simulink model "Proyecto_Global_AyCD_Ultimo"  (R2017b)
settings: Solver=FixedStepAuto  StartTime=0.0  StopTime=inf  FixedStep=0.01  RelTol=1e-3  EnableMultiTasking=on
values from neighbouring files (symbols this model uses):
  AhMax = 1    [datosAyCD.m]
  AtMax = 1    [datosAyCD.m]
  Ba_b = zeros(1,60)    [PD_balanceo_CARGA_GainScheduling.m]
  Ba_h = Mh*n_h*Wpos_h    [PID_izaje_CARGA.m]
  Ba_t = Mt*n_t*Wpos_t    [PID_traslacion_CARRO.m]
  bContenedor = 2.5    [datosAyCD.m]
  bh = bhEq*rh^2/Rd^2    (= 28800)    [datosAyCD.m]
  bt = btEq*rt^2/Rw^2    (= 27000)    [datosAyCD.m]
  bw = 30000    [datosAyCD.m]
  cantidadCarrilesBarco = 9+1    (= 10)    [datosAyCD.m]
  g = 9.80665    [datosAyCD.m]
  hContenedor = 2.5    [datosAyCD.m]
  hLimInf = -17.5-2    (= -19.5)    [datosAyCD.m]
  hLimSup = 40+2    (= 42)    [datosAyCD.m]
  Kd = zeros(1,60)    [PD_balanceo_CARGA_AutoTunning.m]
  Kp = zeros(1,60)    [PD_balanceo_CARGA_AutoTunning.m]
  Ksa_b = zeros(1,60)    [PD_balanceo_CARGA_GainScheduling.m]
  Ksa_h = Mh*n_h*Wpos_h^2    [PID_izaje_CARGA.m]
  Ksa_t = Mt*n_t*Wpos_t^2    [PID_traslacion_CARRO.m]
  Ksia_h = Mh*Wpos_h^3    [PID_izaje_CARGA.m]
  Ksia_t = Mt*Wpos_t^3    [PID_traslacion_CARRO.m]
  Kw = 1800000    [datosAyCD.m]
  l1 = zeros(1,60)    [PD_balanceo_CARGA_AutoTunning.m]
  Mh = (Jd+Jmh*rh^2) / (Rd^2)    (= 48014.2222222)    [datosAyCD.m]
  mlMax = mlMin+48000    (= 65000)    [datosAyCD.m]
  mlVacio = 15000    [datosAyCD.m]
  Mt = mc + (Jw+Jmt*rt^2) / (Rw^2)    (= 59008)    [datosAyCD.m]
  nRand = [14 17 20 22 20 17 14 8 8 8]    [datosAyCD.m]
  Rd = 0.75    [datosAyCD.m]
  rh = 30    [datosAyCD.m]
  rt = 15    [datosAyCD.m]
  Rw = 0.5    [datosAyCD.m]
  Tf = zeros(1,60)    [PD_balanceo_CARGA_AutoTunning.m]
  tLimDer = 50+2    (= 52)    [datosAyCD.m]
  tLimIzq = -30-2    (= -32)    [datosAyCD.m]
  VhMaxC = 1.5    [datosAyCD.m]
  VhMaxV = 3    [datosAyCD.m]
  xCarrilBarco = zeros(1,cantidadCarrilesBarco)    [datosAyCD.m]
  xCarrilMuelle = [-30,-25,-20,-15,-10,-5]    [datosAyCD.m]
  yCarrilBarcoPar = zeros(1,cantidadCarrilesBarco)    [datosAyCD.m]
  ySB = 15    [datosAyCD.m]
  yt0 = 45    [datosAyCD.m]
undefined symbols (not defined in the file or in its folder): carrilObjetivoInput, carrilPartidaInput, lh
libraries: simulink x5
settings Model: Creator=Facundo  LastModifiedBy=Martin Da Corta
settings DataIOCC: LimitDataPoints=on
settings OptimizationCC: LifeSpan=inf
settings DebuggingCC: SFUnexpectedBacktrackingDiag=warning  SFNoUnconditionalDefaultTransitionDiag=warning  SFExecutionAtInitializationDiag=none
settings HardwareCC: ProdBitPerSizeT=32  ProdBitPerPtrDiffT=32  ProdWordSize=32  ProdHWDeviceType=Specified
settings ModelReferenceCC: PropagateSignalLabelsOutOfModel=off
settings RTWCC: TargetLang=C++
settings CodeAppCC: StateflowObjectComments=on
settings GRTTargetCC: TargetLangStandard=C89/C90 (ANSI)  MultiInstanceERTCode=on  CodeInterfacePackaging=C++ class
settings ConfigComp: CovMetricSettings=dw  CovHtmlReporting=on  CovSaveCumulativeToWorkspaceVar=on  CovSaveSingleToWorkspaceVar=on  CovExternalEMLEnable=off

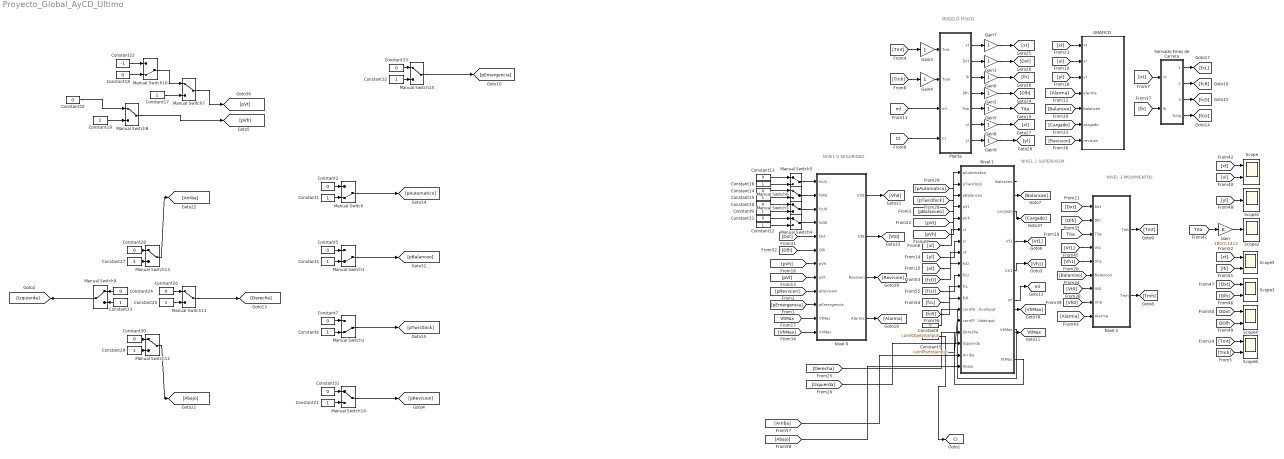
== system Proyecto_Global_AyCD_Ultimo ==
  note: MODELO
      | FÍSICO
  note: NIVEL 2
      | MOVIMIENTOS
  note: NIVEL 0
      | SEGURIDAD
  note: NIVEL 1
      | SUPERVISOR
  " Planta" : Subsystem
  Constant{1,4,6,9,12,15..17,19,21,23,25,27,29,32} (15 alike) : Constant  OutDataTypeStr=boolean
  Constant{2,5,7,10..11,13..14,18,20,24,26,28,30..31,33} (15 alike) : Constant  Value=0  OutDataTypeStr=boolean
  Constant22 : Constant  Value=-1  OutDataTypeStr=boolean
  Constant3 : Constant  Value=carrilPartidaInput
  Constant8 : Constant  Value=carrilObjetivoInput
  GRAFICO : Stateflow chart  TreatAsAtomicUnit=on
  Gain : Gain  Gain=180/3.1415
  Gain{1..9} (9 alike) : Gain
  Manual Switch{,1..2,10} (4 alike) : ManualSwitch  CurrentSetting=0
  Manual Switch{3..9,11..15} (12 alike) : ManualSwitch
  Nivel 0 : Stateflow chart  TreatAsAtomicUnit=on
  Nivel 1 : Stateflow chart  TreatAsAtomicUnit=on
  Nivel 2 : Subsystem
  Scope{,3..6} (5 alike) : Scope  NumInputPorts=2
  Scope1 : Scope
  Scope2 : Scope
  Sensado Fines de Carrera : Subsystem
  tag scope: CI=global, Tita=global, VtMax=global, ml=global
  wires:
  [xt] -> Sensado Fines de Carrera/1(xt)
  [lh] -> Sensado Fines de Carrera/2(lh)
  Sensado Fines de Carrera/2(fcRight) -> [fcR]
  Sensado Fines de Carrera/1(fcLeft) -> [fcL]
  Sensado Fines de Carrera/3(fcDown) -> [fcD]
  Sensado Fines de Carrera/4(fcUp) -> [fcU]
  Gain5/1 -> [Tita]
  Gain2/1 -> [Dlh]
  " Planta"/4(Dlh) -> Gain2/1
  " Planta"/5(Tita) -> Gain5/1
  [Tmh] -> Gain4/1
  Gain3/1 -> " Planta"/1(Tmt)
  [Tmt] -> Gain3/1
  " Planta"/6(xl) -> Gain8/1
  Gain6/1 -> [lh]
  " Planta"/1(xt) -> Gain7/1
  " Planta"/3(lh) -> Gain6/1
  Gain4/1 -> " Planta"/2(Tmh)
  Gain1/1 -> [Dxt]
  " Planta"/7(yl) -> Gain9/1
  " Planta"/2(Dxt) -> Gain1/1
  Gain7/1 -> [xt]
  Gain8/1 -> [xl]
  Gain9/1 -> [yl]
  [ml] -> " Planta"/3(ml)
  [pTwistlock] -> Nivel 1/2(pTwistlock)
  Nivel 1/1(Balanceo) -> [Balanceo]
  Nivel 1/3(Vt1) -> [Vt1]
  Nivel 1/4(Vh1) -> [Vh1]
  Constant8/1 -> Nivel 1/13(carrilObjetivoInput)
  [pVt] -> Nivel 1/4(pVt)
  [pVh] -> Nivel 1/5(pVh)
  Nivel 1/5(ml) -> [ml]
  Constant3/1 -> Nivel 1/14(carrilPartidaInput), [CI]
  [pAutomatico] -> Nivel 1/1(pAutomatico)
  [pBalanceo] -> Nivel 1/3(pBalanceo)
  [Vt0] -> Nivel 2/7(Vt0)
  [Vh1] -> Nivel 2/5(Vh1)
  [Alarma] -> Nivel 2/9(Alarma)
  [Dlh] -> Nivel 2/2(Dlh)
  [Vh0] -> Nivel 2/8(Vh0)
  Nivel 2/2(Tmh) -> [Tmh]
  [Dxt] -> Nivel 2/1(Dxt)
  Nivel 2/1(Tmt) -> [Tmt]
  [Vt1] -> Nivel 2/4(Vt1)
  [Balanceo] -> Nivel 2/6(Balanceo)
  [Tita] -> Nivel 2/3(Tita)
  [CI] -> " Planta"/4(CI)
  Nivel 0/2(Vt0) -> [Vt0]
  Nivel 0/1(Vh0) -> [Vh0]
  [pEmergencia] -> Nivel 0/10(pEmergencia)
  Manual Switch3/1 -> Nivel 0/3(fcU0)
  Nivel 0/4(Alarma) -> [Alarma]
  Manual Switch6/1 -> Nivel 0/2(fcR0)
  Manual Switch4/1 -> Nivel 0/4(fcD0)
  Manual Switch5/1 -> Nivel 0/1(fcL0)
  [Dxt] -> Nivel 0/5(Dxt)
  [Dlh] -> Nivel 0/6(Dlh)
  [pRevision] -> Nivel 0/9(pRevision)
  Manual Switch2/1 -> [pTwistlock]
  Manual Switch/1 -> [pAutomatico]
  Constant2/1 -> Manual Switch/1
  Manual Switch1/1 -> [pBalanceo]
  Constant5/1 -> Manual Switch1/1
  Constant1/1 -> Manual Switch/2
  Constant4/1 -> Manual Switch1/2
  Constant6/1 -> Manual Switch2/2
  Constant7/1 -> Manual Switch2/1
  Nivel 1/2(cargado) -> [Cargado]
  [xt] -> GRAFICO/1(xt)
  [xl] -> GRAFICO/2(xl)
  [yl] -> GRAFICO/3(yl)
  [Balanceo] -> GRAFICO/5(balanceo)
  [Cargado] -> GRAFICO/6(cargado)
  [yl] -> Nivel 1/7(yl)
  [xl] -> Nivel 1/6(xl)
  [xt] -> Nivel 1/8(xt)
  [Alarma] -> GRAFICO/4(alarma)
  [pVt] -> Nivel 0/8(pVt)
  [pVh] -> Nivel 0/7(pVh)
  Nivel 1/6(VhMax) -> [VhMax]
  Nivel 1/7(VtMax) -> [VtMax]
  [VtMax] -> Nivel 0/11(VtMax)
  [VhMax] -> Nivel 0/12(VhMax)
  [Revision] -> GRAFICO/7(revision)
  Nivel 0/3(Revision) -> [Revision]
  [xt] -> Scope/1
  [xl] -> Scope/2
  [yl] -> Scope1/1
  Gain/1 -> Scope2/1
  [Tita] -> Gain/1
  [Dxt] -> Scope3/1
  [Dlh] -> Scope3/2
  [DDxt] -> Scope4/1
  [DDlh] -> Scope4/2
  [lh] -> Scope5/2
  [xt] -> Scope5/1
  [fcL] -> Nivel 1/11(fcL)
  [fcR] -> Nivel 1/12(fcR)
  [fcU] -> Nivel 1/10(fcU)
  [fcD] -> Nivel 1/9(fcD)
  Constant9/1 -> Manual Switch3/2
  Constant10/1 -> Manual Switch3/1
  Constant11/1 -> Manual Switch4/1
  Constant12/1 -> Manual Switch4/2
  Constant13/1 -> Manual Switch5/1
  Constant15/1 -> Manual Switch6/2
  Constant16/1 -> Manual Switch5/2
  Constant14/1 -> Manual Switch6/1
  [Tmh] -> Scope6/2
  [Tmt] -> Scope6/1
  Manual Switch7/1 -> [pVt]
  Constant17/1 -> Manual Switch7/2
  Constant19/1 -> Manual Switch8/2
  Manual Switch8/1 -> [pVh]
  Constant20/1 -> Manual Switch8/1
  Constant18/1 -> Manual Switch10/2
  Constant22/1 -> Manual Switch10/1
  Manual Switch10/1 -> Manual Switch7/1
  Manual Switch9/1 -> [Izquierda]
  Constant24/1 -> Manual Switch9/1
  Constant23/1 -> Manual Switch9/2
  Manual Switch11/1 -> [Derecha]
  Constant25/1 -> Manual Switch11/2
  Constant26/1 -> Manual Switch11/1
  [Derecha] -> Nivel 1/15(Derecha)
  [Izquierda] -> Nivel 1/16(Izquierda)
  Manual Switch12/1 -> [Abajo]
  Manual Switch13/1 -> [Arriba]
  Constant29/1 -> Manual Switch12/2
  Constant30/1 -> Manual Switch12/1
  Constant27/1 -> Manual Switch13/2
  Constant28/1 -> Manual Switch13/1
  [Arriba] -> Nivel 1/17(Arriba)
  [Abajo] -> Nivel 1/18(Abajo)
  Constant21/1 -> Manual Switch14/2
  Constant31/1 -> Manual Switch14/1
  Manual Switch14/1 -> [pRevision]
  Constant33/1 -> Manual Switch15/1
  Constant32/1 -> Manual Switch15/2
  Manual Switch15/1 -> [pEmergencia]

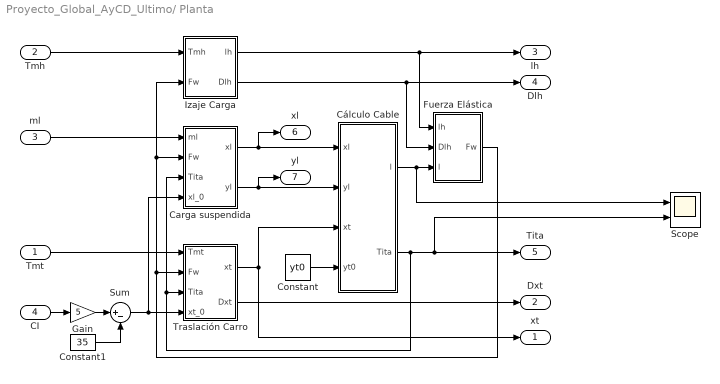
== system Proyecto_Global_AyCD_Ultimo/ Planta ==
  Tmt : Inport
  Tmh : Inport  Port=2
  ml : Inport  Port=3
  CI : Inport  Port=4
  Carga suspendida : Subsystem
  Constant : Constant  Value=yt0
  Constant1 : Constant  Value=35
  Cálculo Cable : MATLAB Function  TreatAsAtomicUnit=on
  Fuerza Elástica : Subsystem
  Gain : Gain  Gain=5
  Izaje Carga : Subsystem
  Scope : Scope  NumInputPorts=2
  Sum : Sum  Inputs=|+-
  Traslación Carro : Subsystem
  xt : Outport
  Dxt : Outport  Port=2
  lh : Outport  Port=3
  Dlh : Outport  Port=4
  Tita : Outport  Port=5
  xl : Outport  Port=6
  yl : Outport  Port=7
  wires:
  Carga suspendida/1(xl) -> xl/1, Cálculo Cable/1(xl)
  Tmh/1 -> Izaje Carga/1(Tmh)
  Constant/1 -> Cálculo Cable/4(yt0)
  Cálculo Cable/2(Tita) -> Scope/2, Tita/1, Carga suspendida/3(Tita), Traslación Carro/3(Tita)
  Fuerza Elástica/1(Fw) -> Izaje Carga/2(Fw), Carga suspendida/2(Fw), Traslación Carro/2(Fw)
  Tmt/1 -> Traslación Carro/1(Tmt)
  Traslación Carro/1(xt) -> xt/1, Cálculo Cable/3(xt)
  Izaje Carga/1(lh) -> lh/1, Fuerza Elástica/1(lh)
  Carga suspendida/2(yl) -> yl/1, Cálculo Cable/2(yl)
  Traslación Carro/2(Dxt) -> Dxt/1
  Izaje Carga/2(Dlh) -> Dlh/1, Fuerza Elástica/2(Dlh)
  ml/1 -> Carga suspendida/1(ml)
  CI/1 -> Gain/1
  Sum/1 -> Carga suspendida/4(xl_0), Traslación Carro/4(xt_0)
  Gain/1 -> Sum/1
  Constant1/1 -> Sum/2
  Cálculo Cable/1(l) -> Scope/1, Fuerza Elástica/3(l)

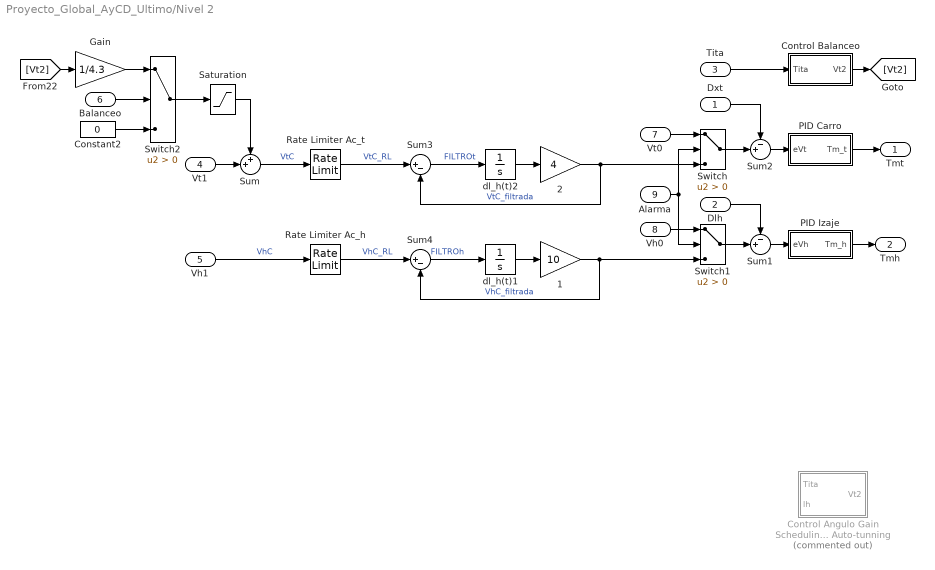
== system Proyecto_Global_AyCD_Ultimo/Nivel 2 ==
  Dxt : Inport
  Dlh : Inport  Port=2
  Tita : Inport  Port=3
  Vt1 : Inport  Port=4
  Vh1 : Inport  Port=5
  Balanceo : Inport  Port=6
  Vt0 : Inport  Port=7
  Vh0 : Inport  Port=8
  Alarma : Inport  Port=9
  1 : Gain  Gain=10
  2 : Gain  Gain=4
  Constant2 : Constant  Value=0
  Control Angulo Gain Scheduling Auto-tunning : Subsystem  Commented=on
  Control Balanceo : Subsystem
  Gain : Gain  Gain=1/4.3
  PID Carro : Subsystem
  PID Izaje : Subsystem
  Rate Limiter Ac_h : RateLimiter  RisingSlewLimit=AhMax  FallingSlewLimit=-AhMax
  Rate Limiter Ac_t : RateLimiter  RisingSlewLimit=AtMax  FallingSlewLimit=-AtMax
  "Saturation " : Saturate  UpperLimit=5  LowerLimit=-5
  Sum : Sum  Inputs=++|
  Sum1 : Sum  Inputs=-+|
  Sum2 : Sum  Inputs=-+|
  Sum3 : Sum  Inputs=|+-
  Sum4 : Sum  Inputs=|+-
  Switch : Switch  Criteria=u2 > Threshold
  Switch1 : Switch  Criteria=u2 > Threshold
  Switch2 : Switch  Criteria=u2 > Threshold
  dl_h(t)1 : Integrator
  dl_h(t)2 : Integrator
  Tmt : Outport
  Tmh : Outport  Port=2
  wires:
  Control Balanceo/1(Vt2) -> [Vt2]
  PID Carro/1(Tm_t) -> Tmt/1
  PID Izaje/1(Tm_h) -> Tmh/1
  Dxt/1 -> Sum2/1
  Vt1/1 -> Sum/2
  Balanceo/1 -> Switch2/2
  Constant2/1 -> Switch2/3
  Switch2/1 -> "Saturation "/1
  "Saturation "/1 -> Sum/1
  Sum/1 -> Rate Limiter Ac_t/1  "VtC"
  Vt0/1 -> Switch/1
  Alarma/1 -> Switch/2, Switch1/2
  Vh0/1 -> Switch1/1
  Switch/1 -> Sum2/2
  Sum2/1 -> PID Carro/1(eVt)
  Sum1/1 -> PID Izaje/1(eVh)
  Switch1/1 -> Sum1/2
  Dlh/1 -> Sum1/1
  dl_h(t)2/1 -> 2/1
  Sum3/1 -> dl_h(t)2/1  "FILTROt"
  2/1 -> Switch/3, Sum3/2  "VtC_filtrada"
  Rate Limiter Ac_t/1 -> Sum3/1  "VtC_RL"
  Rate Limiter Ac_h/1 -> Sum4/1  "VhC_RL"
  1/1 -> Switch1/3, Sum4/2  "VhC_filtrada"
  Sum4/1 -> dl_h(t)1/1  "FILTROh"
  dl_h(t)1/1 -> 1/1
  [Vt2] -> Gain/1
  Gain/1 -> Switch2/1
  Tita/1 -> Control Balanceo/1(Tita)
  Vh1/1 -> Rate Limiter Ac_h/1  "VhC"

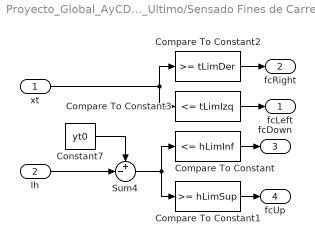
== system Proyecto_Global_AyCD_Ultimo/Sensado Fines de Carrera ==
  xt : Inport
  lh : Inport  Port=2
  Compare To Constant : simulink/Logic and Bit Operations/Compare To Constant  relop=<=  const=hLimInf  OutDataTypeStr=uint8
  Compare To Constant1 : simulink/Logic and Bit Operations/Compare To Constant  relop=>=  const=hLimSup  OutDataTypeStr=uint8
  Compare To Constant2 : simulink/Logic and Bit Operations/Compare To Constant  relop=>=  const=tLimDer  OutDataTypeStr=uint8
  Compare To Constant3 : simulink/Logic and Bit Operations/Compare To Constant  relop=<=  const=tLimIzq  OutDataTypeStr=uint8
  Constant7 : Constant  Value=yt0
  Sum4 : Sum  Inputs=+-|
  fcLeft : Outport
  fcRight : Outport  Port=2
  fcDown : Outport  Port=3
  fcUp : Outport  Port=4
  wires:
  lh/1 -> Sum4/2
  Constant7/1 -> Sum4/1
  Sum4/1 -> Compare To Constant/1, Compare To Constant1/1
  Compare To Constant2/1 -> fcRight/1
  Compare To Constant/1 -> fcDown/1
  Compare To Constant1/1 -> fcUp/1
  Compare To Constant3/1 -> fcLeft/1
  xt/1 -> Compare To Constant3/1, Compare To Constant2/1

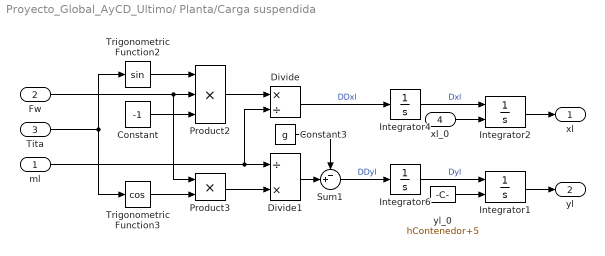
== system Proyecto_Global_AyCD_Ultimo/ Planta/Carga suspendida ==
  ml : Inport
  Fw : Inport  Port=2
  Tita : Inport  Port=3
  xl_0 : Inport  Port=4
  Constant : Constant  Value=-1
  Constant3 : Constant  Value=g
  Divide : Product  Inputs=*/
  Divide1 : Product  Inputs=/*
  Integrator1 : Integrator  InitialConditionSource=external
  Integrator2 : Integrator  InitialConditionSource=external
  Integrator4 : Integrator
  Integrator6 : Integrator
  Product2 : Product  Inputs=3
  Product3 : Product
  Sum1 : Sum  Inputs=-+|
  Trigonometric Function2 : Trigonometry
  Trigonometric Function3 : Trigonometry  Operator=cos
  yl_0 : Constant  Value=hContenedor+5
  xl : Outport
  yl : Outport  Port=2
  wires:
  Sum1/1 -> Integrator6/1  "DDyl"
  Constant3/1 -> Sum1/1
  Integrator2/1 -> xl/1
  Integrator6/1 -> Integrator1/1  "Dyl"
  Divide1/1 -> Sum1/2
  Product3/1 -> Divide1/2
  Product2/1 -> Divide/1
  Fw/1 -> Product3/1, Product2/2
  Trigonometric Function2/1 -> Product2/1
  Trigonometric Function3/1 -> Product3/2
  Tita/1 -> Trigonometric Function2/1, Trigonometric Function3/1
  Constant/1 -> Product2/3
  ml/1 -> Divide/2, Divide1/1
  Divide/1 -> Integrator4/1  "DDxl"
  xl_0/1 -> Integrator2/2
  Integrator4/1 -> Integrator2/1  "Dxl"
  Integrator1/1 -> yl/1
  yl_0/1 -> Integrator1/2

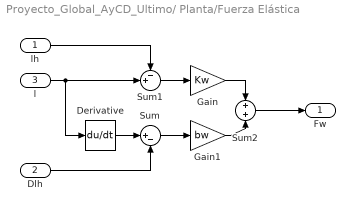
== system Proyecto_Global_AyCD_Ultimo/ Planta/Fuerza Elástica ==
  lh : Inport
  Dlh : Inport  Port=2
  l : Inport  Port=3
  Derivative : Derivative
  Gain : Gain  Gain=Kw
  Gain1 : Gain  Gain=bw
  Sum : Sum  Inputs=|+-
  Sum1 : Sum  Inputs=-+|
  Sum2 : Sum  Inputs=+|+
  Fw : Outport
  wires:
  Dlh/1 -> Sum/2
  lh/1 -> Sum1/1
  Derivative/1 -> Sum/1
  Sum1/1 -> Gain/1
  Sum/1 -> Gain1/1
  l/1 -> Derivative/1, Sum1/2
  Sum2/1 -> Fw/1
  Gain1/1 -> Sum2/2
  Gain/1 -> Sum2/1

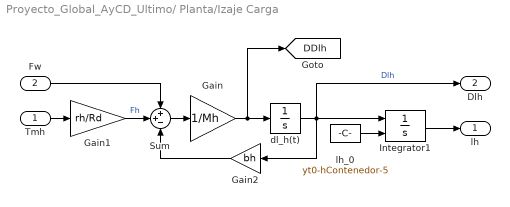
== system Proyecto_Global_AyCD_Ultimo/ Planta/Izaje Carga ==
  Tmh : Inport
  Fw : Inport  Port=2
  Gain : Gain  Gain=1/Mh
  Gain1 : Gain  Gain=rh/Rd
  Gain2 : Gain  Gain=bh
  Integrator1 : Integrator  InitialConditionSource=external
  Sum : Sum  Inputs=++-
  dl_h(t) : Integrator
  lh_0 : Constant  Value=yt0-hContenedor-5
  lh : Outport
  Dlh : Outport  Port=2
  tag scope: DDlh=global
  wires:
  Fw/1 -> Sum/1
  Tmh/1 -> Gain1/1
  Integrator1/1 -> lh/1
  Gain1/1 -> Sum/2  "Fh"
  Gain2/1 -> Sum/3
  Sum/1 -> Gain/1
  dl_h(t)/1 -> Dlh/1, Integrator1/1, Gain2/1  "Dlh"
  lh_0/1 -> Integrator1/2
  Gain/1 -> dl_h(t)/1, [DDlh]

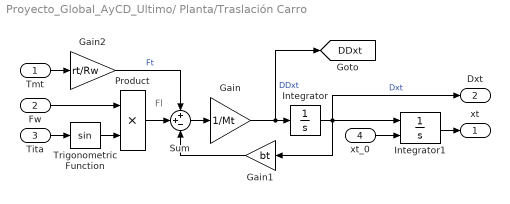
== system Proyecto_Global_AyCD_Ultimo/ Planta/Traslación Carro ==
  note: Fl
  Tmt : Inport
  Fw : Inport  Port=2
  Tita : Inport  Port=3
  xt_0 : Inport  Port=4
  Gain : Gain  Gain=1/Mt
  Gain1 : Gain  Gain=bt
  Gain2 : Gain  Gain=rt/Rw
  Integrator : Integrator
  Integrator1 : Integrator  InitialConditionSource=external
  Product : Product
  Sum : Sum  Inputs=++-
  Trigonometric Function : Trigonometry
  xt : Outport
  Dxt : Outport  Port=2
  tag scope: DDxt=global
  wires:
  Gain/1 -> [DDxt], Integrator/1  "DDxt"
  Product/1 -> Sum/2
  Sum/1 -> Gain/1
  Gain1/1 -> Sum/3
  Tmt/1 -> Gain2/1
  Gain2/1 -> Sum/1  "Ft"
  Trigonometric Function/1 -> Product/2
  Tita/1 -> Trigonometric Function/1
  Fw/1 -> Product/1
  Integrator/1 -> Gain1/1, Dxt/1, Integrator1/1  "Dxt"
  xt_0/1 -> Integrator1/2
  Integrator1/1 -> xt/1

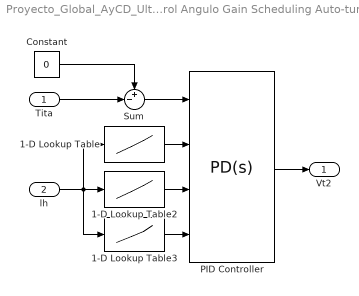
== system Proyecto_Global_AyCD_Ultimo/Nivel 2/Control Angulo Gain Scheduling Auto-tunning ==
  Tita : Inport
  lh : Inport  Port=2
  1-D Lookup Table : Lookup_n-D  NumberOfTableDimensions=1  BreakpointsForDimension1=l1  Table=Kp  InternalRulePriority=Speed  RndMeth=Simplest  InputSameDT=on
  1-D Lookup Table2 : Lookup_n-D  NumberOfTableDimensions=1  BreakpointsForDimension1=l1  Table=Kd  InternalRulePriority=Speed  RndMeth=Simplest  InputSameDT=on
  1-D Lookup Table3 : Lookup_n-D  NumberOfTableDimensions=1  BreakpointsForDimension1=l1  Table=Tf  InternalRulePriority=Speed  RndMeth=Simplest  InputSameDT=on
  Constant : Constant  Value=0
  PID Controller : simulink/Continuous/PID Controller  Controller=PD  TimeDomain=Continuous-time  SampleTime=-1  IntegratorMethod=Forward Euler  FilterMethod=Forward Euler  Form=Parallel  UseFilter=on  ControllerParametersSource=external  P=1  I=1  D=0  N=100  InitialConditionSource=internal  InitialConditionForIntegrator=0  InitialConditionForFilter=0  ExternalReset=none  LimitOutput=off  UpperSaturationLimit=inf  LowerSaturationLimit=-inf  LinearizeAsGain=on  AntiWindupMode=none  Kb=1  TrackingMode=off  Kt=1  PParamMin=[]  PParamMax=[]  IParamMin=[]  IParamMax=[]  DParamMin=[]  DParamMax=[]  NParamMin=[]  NParamMax=[]  KbParamMin=[]  KbParamMax=[]  KtParamMin=[]  KtParamMax=[]  POutMin=[]  POutMax=[]  IOutMin=[]  IOutMax=[]  DOutMin=[]  DOutMax=[]  NOutMin=[]  NOutMax=[]  KbOutMin=[]  KbOutMax=[]  KtOutMin=[]  KtOutMax=[]  IntegratorOutMin=[]  IntegratorOutMax=[]  FilterOutMin=[]  FilterOutMax=[]  SumOutMin=[]  SumOutMax=[]  SumI1OutMin=[]  SumI1OutMax=[]  SumI2OutMin=[]  SumI2OutMax=[]  SumI3OutMin=[]  SumI3OutMax=[]  SumDOutMin=[]  SumDOutMax=[]  SaturationOutMin=[]  SaturationOutMax=[]  IntegratorContinuousStateAttributes=''  IntegratorStateMustResolveToSignalObject=off  IntegratorRTWStateStorageClass=Auto  FilterContinuousStateAttributes=''  FilterStateMustResolveToSignalObject=off  FilterRTWStateStorageClass=Auto  DifferentiatorICPrevScaledInput=0  DifferentiatorOutMin=[]  DifferentiatorOutMax=[]  FilterDiffOutCoefMin=[]  FilterDiffOutCoefMax=[]  SumDenOutMin=[]  SumDenOutMax=[]  SumNumOutMin=[]  SumNumOutMax=[]  ReciprocalOutMin=[]  ReciprocalOutMax=[]  DivideOutMin=[]  DivideOutMax=[]  TunerSelectOption=Transfer Function Based (PID Tuner App)
  Sum : Sum  Inputs=+-|
  Vt2 : Outport
  wires:
  Tita/1 -> Sum/2
  1-D Lookup Table/1 -> PID Controller/2
  1-D Lookup Table2/1 -> PID Controller/3
  1-D Lookup Table3/1 -> PID Controller/4
  Sum/1 -> PID Controller/1
  PID Controller/1 -> Vt2/1
  Constant/1 -> Sum/1
  lh/1 -> 1-D Lookup Table3/1, 1-D Lookup Table/1, 1-D Lookup Table2/1

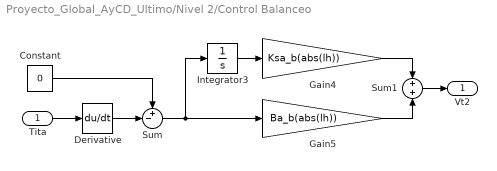
== system Proyecto_Global_AyCD_Ultimo/Nivel 2/Control Balanceo ==
  Tita : Inport
  Constant : Constant  Value=0
  Derivative : Derivative
  Gain4 : Gain  Gain=Ksa_b(abs(lh))
  Gain5 : Gain  Gain=Ba_b(abs(lh))
  Integrator3 : Integrator
  Sum : Sum  Inputs=+-|
  Sum1 : Sum  Inputs=+|+
  Vt2 : Outport
  wires:
  Integrator3/1 -> Gain4/1
  Constant/1 -> Sum/1
  Tita/1 -> Derivative/1
  Derivative/1 -> Sum/2
  Gain4/1 -> Sum1/1
  Gain5/1 -> Sum1/2
  Sum1/1 -> Vt2/1
  Sum/1 -> Integrator3/1, Gain5/1

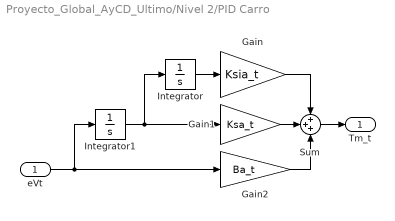
== system Proyecto_Global_AyCD_Ultimo/Nivel 2/PID Carro ==
  eVt : Inport
  Gain : Gain  Gain=Ksia_t
  Gain1 : Gain  Gain=Ksa_t
  Gain2 : Gain  Gain=Ba_t
  Integrator : Integrator
  Integrator1 : Integrator
  Sum : Sum  Inputs=+++
  Tm_t : Outport
  wires:
  Gain2/1 -> Sum/3
  Gain/1 -> Sum/1
  Sum/1 -> Tm_t/1
  Integrator1/1 -> Integrator/1, Gain1/1
  Integrator/1 -> Gain/1
  Gain1/1 -> Sum/2
  eVt/1 -> Integrator1/1, Gain2/1

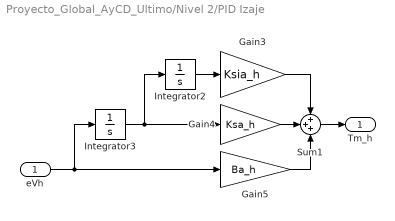
== system Proyecto_Global_AyCD_Ultimo/Nivel 2/PID Izaje ==
  eVh : Inport
  Gain3 : Gain  Gain=Ksia_h
  Gain4 : Gain  Gain=Ksa_h
  Gain5 : Gain  Gain=Ba_h
  Integrator2 : Integrator
  Integrator3 : Integrator
  Sum1 : Sum  Inputs=+++
  Tm_h : Outport
  wires:
  Gain5/1 -> Sum1/3
  Gain3/1 -> Sum1/1
  Sum1/1 -> Tm_h/1
  Integrator3/1 -> Integrator2/1, Gain4/1
  Integrator2/1 -> Gain3/1
  Gain4/1 -> Sum1/2
  eVh/1 -> Integrator3/1, Gain5/1

== stateflow chart Proyecto_Global_AyCD_Ultimo/Nivel 1 ==
  state SPREADER [parallel]
    entry: lado = 0;
    settings: executionOrder=1
    state CARGADO
      entry:
      calculaCarrilActual();
      VhMax=VhMaxC;
      ml=mlMax; cargado=1;
      calculaG();
    state VACIO
      entry:
      calculaCarrilActual();
      VhMax=VhMaxV;
      ml=mlVacio; cargado=0;
      calculaG();
    (default) -> CARGADO
    VACIO -> CARGADO : [pTwistlock==1]
    CARGADO -> VACIO : [pTwistlock==0]
  state LADO [parallel]
    settings: executionOrder=2
    state BARCO
      entry: lado=1;
    state MUELLE
      entry: lado=0;
    (default) -> MUELLE
    MUELLE -> BARCO : [xt>=0]
    BARCO -> MUELLE : [xt<0]
  state BALANCEO [parallel]
    settings: executionOrder=3
    state DESACTIVADO
      entry:
      Balanceo=0;
    state ACTIVADO
      entry:
      Balanceo=1;
    (default) -> ACTIVADO
    DESACTIVADO -> ACTIVADO : [pBalanceo==1]
    ACTIVADO -> DESACTIVADO : [pBalanceo==0]
  state FUNCIONAMIENTO [parallel]
    entry:
    yCarrilBarco=yCarrilBarcoPar;
    VtMax = 4;
    Vh1=0;
    Vt1=0;
    settings: executionOrder=4
    state AUTOMATICO
      state MUELLE_A_BARCO
        entry:
        carrilObjetivo = carrilObjetivoInput+1; calculaCarrilActual(); carrilPartida = carrilActual; calculaTrayectoria();
        finTida=0;
        finHida=0;
        state TRASL_IZAJE_ASC_A_BARCO
          entry:
          Vt1 = VtMax;
          during:
          calculaVt1();
        state IZAJE_INICIAL_A_BARCO
          entry:
          Vt1 = 0;
          Vh1=-VhMax;
        state TRASLACION_A_BARCO
          entry:
          Vh1 = 0;
          during:
          calculaVt1();
        state TRASL_IZAJE_DESC_A_BARCO
          entry:
          Vh1=VhMax;
          during:
          calculaVt1();
          calculaVh1();
        state STOP_A_BARCO
          entry:
          finTida=1;
          finHida=1;
        (default) -> IZAJE_INICIAL_A_BARCO
        IZAJE_INICIAL_A_BARCO -> TRASL_IZAJE_ASC_A_BARCO : [yl>(y_inicial1-1)]
        TRASL_IZAJE_ASC_A_BARCO -> TRASLACION_A_BARCO : [yl>(Ymax-1.5)]
        TRASLACION_A_BARCO -> TRASL_IZAJE_DESC_A_BARCO [order 1] : [xl>=(xYmax+x_inicial1)]
        TRASLACION_A_BARCO -> TRASL_IZAJE_DESC_A_BARCO [order 2] : [xl>(xObjetivo-2)]
        TRASL_IZAJE_DESC_A_BARCO -> STOP_A_BARCO : [(Vt1==0)&&Vh1==0]
      state FIN_IDA
      state FIN_VUELTA
      state BARCO_A_MUELLE
        entry:
        calculaCarrilActual(); carrilObjetivo = carrilActual; carrilPartida   = carrilPartidaInput; calculaTrayectoria_2();
        finTvuelta = 0;finHvuelta = 0;
        state TRASL_IZAJE_ASC_A_MUELLE
          entry:
          Vt1 = -VtMax;
          during:
          calculaVt1_2();
        state IZAJE_INICIAL_A_MUELLE
          entry:
          Vt1 = 0;
          Vh1=-VhMax;
        state TRASLACION_A_MUELLE
          entry:
          Vh1 = 0;
          during:
          calculaVt1_2();
        state TRASL_IZAJE_DESC_MUELLE
          entry:
          Vh1=VhMax;
          during:
          calculaVt1_2();
          calculaVh1_2();
        state STOP_MUELLE
          entry:
          finTvuelta=1;
          finHvuelta=1;
        (default) -> IZAJE_INICIAL_A_MUELLE
        IZAJE_INICIAL_A_MUELLE -> TRASL_IZAJE_ASC_A_MUELLE : [yl>(y_inicial2+yObjetivo)]
        TRASL_IZAJE_ASC_A_MUELLE -> TRASLACION_A_MUELLE : [yl>(Ymax-1.5)]
        TRASLACION_A_MUELLE -> TRASL_IZAJE_DESC_MUELLE [order 1] : [xl<=(xPartida+2)]
        TRASLACION_A_MUELLE -> TRASL_IZAJE_DESC_MUELLE [order 2] : [xl<=(xYmax-x_inicial2)]
        TRASL_IZAJE_DESC_MUELLE -> STOP_MUELLE : [(Vt1==0)&&Vh1==0]
      (junction 527) -> MUELLE_A_BARCO [order 1] : [lado==0]
      MUELLE_A_BARCO -> FIN_IDA : [(finTida==1)&&(finHida==1)]
      FIN_VUELTA -> MUELLE_A_BARCO : [(pAutomatico==1)]
      (default) -> (junction 527)
      (junction 527) -> BARCO_A_MUELLE [order 2] : [lado==1]
      FIN_IDA -> BARCO_A_MUELLE : [(pAutomatico==1)]
      BARCO_A_MUELLE -> FIN_VUELTA : [(finTvuelta==1)&(finHvuelta==1)]
    state MANUAL
      state TRASLACION [parallel]
        entry:
        Vh1=0;
        settings: executionOrder=1
        state STOP
          entry:
          Vt1=0;
        state A_MUELLE
          entry:
          Vh1 = 0;
          Vt1=-VtMax/5;
        state A_BARCO
          entry:
          Vh1 = 0;
          Vt1=VtMax/5;
        FUNCIONAMIENTO.MANUAL.TRASLACION.STOP -> A_BARCO [order 2] : [Derecha==1]
        (default) -> FUNCIONAMIENTO.MANUAL.TRASLACION.STOP
        FUNCIONAMIENTO.MANUAL.TRASLACION.STOP -> A_MUELLE [order 1] : [Izquierda==1]
        A_MUELLE -> FUNCIONAMIENTO.MANUAL.TRASLACION.STOP : [Izquierda==0]
        A_BARCO -> FUNCIONAMIENTO.MANUAL.TRASLACION.STOP : [Derecha==0]
      state IZAJE [parallel]
        entry:
        Vt1=0;
        settings: executionOrder=2
        state DESCENSO
          entry:
          Vt1 = 0;
          Vh1=VtMax/5;
        state ASCENSO
          entry:
          Vt1 = 0;
          Vh1=-VtMax/5;
        state STOP
          entry:
          Vh1=0;
        FUNCIONAMIENTO.MANUAL.IZAJE.STOP -> ASCENSO [order 2] : [Arriba==1]
        (default) -> FUNCIONAMIENTO.MANUAL.IZAJE.STOP
        FUNCIONAMIENTO.MANUAL.IZAJE.STOP -> DESCENSO [order 1] : [Abajo==1]
        DESCENSO -> FUNCIONAMIENTO.MANUAL.IZAJE.STOP : [Abajo==0]
        ASCENSO -> FUNCIONAMIENTO.MANUAL.IZAJE.STOP : [Arriba==0]
    state FIN_CARRERA
      entry:
      Vt1=0; Vh1=0;
      during:
      calculaVt1_manual();
      calculaVh1_manual();
    (default) -> MANUAL
    MANUAL -> AUTOMATICO [order 1] : [pAutomatico==1]
    AUTOMATICO -> MANUAL [order 5] : [pAutomatico==0]
    AUTOMATICO -> MANUAL [order 4] : [ (pVh>0.2) || (pVh<-0.2) ]
    AUTOMATICO -> MANUAL [order 1] : [ (pVt>0.2) || (pVt<-0.2) ]
    FIN_CARRERA -> MANUAL : [fcL==0 && fcU==0 && fcR==0 && fcL==0]
    MANUAL -> FIN_CARRERA [order 3] : [(fcL==1)||(fcR==1)]
    MANUAL -> FIN_CARRERA [order 2] : [(fcU==1)||(fcD==1)]
    AUTOMATICO -> FIN_CARRERA [order 2] : [(fcU==1)||(fcD==1)]
    AUTOMATICO -> FIN_CARRERA [order 3] : [(fcL==1)||(fcR==1)]
  data: Balanceo output; cargado output; pAutomatico input boolean; pTwistlock input boolean; pBalanceo input; pVt input; pVh input; Vt1 output; Vh1 output; ml output; mlMax parameter; VhMaxC parameter; mlVacio parameter; VhMaxV parameter; lado local; y_inicial1 local; Ymax local; xYmax local; yObjetivo local; ySB parameter; yCarrilBarco local; hContenedor parameter; xObjetivo local; xCarrilBarco parameter; xCarrilMuelle parameter; finTida local; finHida local; finTvuelta local; finHvuelta local; carrilObjetivo local uint8; carrilPartida local uint8; x_inicial1 local; xPartida local; yPartida local; y_inicial2 local; x_inicial2 local; bContenedor parameter; nRand parameter; cantidadCarrilesBarco parameter; miCarril local; carrilActual local uint8; xl input; yl input; xt input; VhMax output; VtMax output; yCarrilBarcoPar parameter; iPar local; fcD input; fcU input; fcL input; fcR input; carrilObjetivoInput input uint8; carrilPartidaInput input uint8; Derecha input; Izquierda input; Arriba input; Abajo input
  function calculaVt1_manual:
    | function calculaVt1_manual
    | 
    | if(   ((pVt>0.2)&&(fcR==0)) || ((pVt<-0.2)&&(fcL==0)) )
    |      Vt1 = pVt*VtMax/3;
    | else
    |      Vt1 = 0;
    | end
  function calculaVh1_manual:
    | function calculaVh1_manual %Descenso de ida
    | 
    | if( ((pVh>0.2)&&(fcD==0)) || ((pVh<-0.2)&&(fcU==0)) )
    |     Vh1 = pVh*VhMax/3;
    | else
    |     Vh1 = 0;
    | end
    | 
    | if ( (fcR==0)&&(fcL==0)&&(fcU==0)&&(fcD==0) )
    |     Revision = 0;
    | else 
    |     Revision = 1;
    | end
  function calculaG:
    | function calculaG %Función auxiliar para agregar o quitar contenedor en columna
    |     if(lado==1)
    |         if (cargado==0) 
    | 
    |             x = xCarrilBarco(carrilActual);
    |             y = yCarrilBarco(carrilActual)-5;
    | 
    |             line([x-bContenedor/2 x-bContenedor/2],[y y+hContenedor],'LineWidth',2,'color','red');
    |             line([x-bContenedor/2 x+bContenedor/2],[y+hContenedor y+hContenedor],'LineWidth',2,'color','red');
    |             line([x+bContenedor/2 x+bContenedor/2],[y+hContenedor y],'LineWidth',2,'color','red');
    | 
    |             yCarrilBarco(carrilActual) = y+5+hContenedor;
    | 
    |         elseif (cargado==1) %si estaba DESCARGADO y CARGA
    | 
    |             x = xCarrilBarco(carrilActual);
    |             y = yCarrilBarco(carrilActual)-5;
    | 
    |             line([x-bContenedor/2 x-bContenedor/2],[y-hContenedor y],'LineWidth',2,'color','white');
    |             line([x-bContenedor/2 x+bContenedor/2],[y             y],'LineWidth',2,'color','white');
    |             line([x+bContenedor/2 x+bContenedor/2],[y y-hContenedor],'LineWidth',2,'color','white');
    | 
    |             yCarrilBarco(carrilActual) = y+5-hContenedor;
    |         end
    |         vol=1;
    |     end
    |     if(lado==0)
    |         if (cargado==0) 
    |             
    |             x = xl;
    |             y = yCarrilBarco(carrilActual)-10;
    | 
    |             line([x-bContenedor/2 x-bContenedor/2],[y y+hContenedor],'LineWidth',2,'color','red');
    |             line([x-bContenedor/2 x+bContenedor/2],[y+hContenedor y+hContenedor],'LineWidth',2,'color','red');
    |             line([x+bContenedor/2 x+bContenedor/2],[y+hContenedor y],'LineWidth',2,'color','red');
    | 
    |             yCarrilBarco(carrilActual) = y+5+hContenedor;
    |           
    |         elseif (cargado==1) %si estaba DESCARGADO y CARGA
    | 
    |             x = xl;
    |             y = yl;
    | 
    |             line([x-bContenedor/2 x-bContenedor/2],[y-hContenedor y],'LineWidth',2,'color','white');
    |             line([x-bContenedor/2 x+bContenedor/2],[y             y],'LineWidth',2,'color','white');
    |             line([x+bContenedor/2 x+bContenedor/2],[y y-hContenedor],'LineWidth',2,'color','white');
    | 
    |             yCarrilBarco(carrilActual) = y+5-hContenedor;
    |         end
    |     end
    | end
  function calculaTrayectoria:
    | function calculaTrayectoria
    | 
    | xObjetivo      = xCarrilBarco(carrilObjetivo);
    | xPartida       = xCarrilMuelle(carrilPartida);
    | yObjetivo      = yCarrilBarco(carrilObjetivo)+2; %2 metros más de seguridad
    | numCarrilBarco = [1 2 3 4 5 6 7 8 9 10 11 12 13 14 15 16 17];
    | 
    | %% Ymax
    | %Obstáculo más alto a alcanzar hasta carril objetivo (de más a la DERECHA)
    | xYmax = 0; Ymax  = 15; carrilYmax = 1;
    | for j=1:carrilObjetivo
    |     if (yCarrilBarco(j)>=Ymax)
    |          Ymax = yCarrilBarco(j);
    |         xYmax = xCarrilBarco(j);%%x que se corresponde a la altura ymax
    |         carrilYmax = numCarrilBarco(j);
    |     end
    | end
    | Ymax = Ymax + 2; %2m extra de seguridad
    | if cargado==1   % Suma altura de contenedor si está cargado
    |      Ymax=Ymax+hContenedor;
    | end
    | 
    | %% Izaje inicial
    | xSB = -xCarrilMuelle(carrilPartida); % Distancia desde posición inicial a ubicación de SB
    | deltaYcarril1    = zeros(1,carrilObjetivo);
    | % Barrido de carriles para ver cuál interfiere más en el recorrido
    | for i=1:carrilObjetivo
    |     distanciaXcarril = xSB + xCarrilBarco(i);
    |     tiempoCarril     = distanciaXcarril/VtMax;
    |     distanciaYcarril = tiempoCarril*VhMax;
    |     deltaYcarril1(i) = yCarrilBarco(i)-(distanciaYcarril+hContenedor); %comienza desde hContenedor (cargado o no)
    | end
    | if cargado==1   % Suma altura de contenedor si está cargado (carga debe pasar por arriba de obstáculo)
    |      deltaYcarril1 = deltaYcarril1+hContenedor;
    | end
    | 
    | if isempty(deltaYcarril1)
    |     y_inicial1 = 2;   % y_inicial es el valor de y del primer izaje antes de comenzar la trayectoria
    | else
    |     y_inicial1 = max(deltaYcarril1)+2; %2m extra de seguridad
    | end
    | 
    | if y_inicial1<0 
    |     y_inicial1 = 0;
    | end
    | 
    | % TRASLACIÓN EXCLUSIVA
    | x_inicial1 = 0;
    | carrilesAderecha = carrilObjetivo-carrilYmax;
    |     
    | if ( carrilesAderecha>1 )
    | 
    |     deltaYcarril12    = zeros(1,carrilObjetivo);
    |     for i=1:carrilObjetivo
    |         deltaYcarril12(i)    = -100;
    |     end
    |     % Barrido carriles para ver cual interfiere más en el recorrido
    |     for i=(carrilYmax+1):carrilObjetivo
    |         distanciaXcarril = xCarrilBarco(i)-xYmax;
    |         tiempoCarril     = distanciaXcarril/VtMax;
    |         distanciaYcarril = tiempoCarril*VhMax;
    |         hYcarril         = Ymax - distanciaYcarril;
    |         deltaYcarril12(i)  = yCarrilBarco(i)-hYcarril;
    |     end
    |     
    |     if isempty(deltaYcarril12)
    |         MAXdeltaY = 0;
    |     else
    |         MAXdeltaY = max(deltaYcarril12);
    |     end
    |     
    |     deltaYdeseada = 3; %2.5m de seguridad
    |     if cargado==1   % Suma altura de contenedor si está cargado
    |         deltaYdeseada = deltaYdeseada+hContenedor;
    |     end
    |     
    |     deltaReal = deltaYdeseada+MAXdeltaY;
    |     if(deltaReal<0)
    |         deltaReal=0;
    |     end
    |         
    |     tMAXdeltaY = deltaReal/VhMax;
    |     distanciatMAX = tMAXdeltaY*VtMax;
    |     x_inicial1 = distanciatMAX;
    | 
    | end
    | 
    | if ( (carrilesAderecha==1) ) 
    |     x_inicial1 = 4;
    | end
    | 
    | if ( (carrilesAderecha==0) && (xYmax==xObjetivo) )
    |     x_inicial1 = -0.75;
    | end
    | 
    | if cargado==1   % Suma altura de contenedor si está cargado
    |      yObjetivo = yObjetivo+hContenedor;
    | end
    | 
    | % xObjetivo
    | % xPartida
    | % yObjetivo 
    | % Ymax
    | % xYmax
    | % carrilYmax
    | % y_inicial1
    | % x_inicial1
  function calculaVt1:
    | function calculaVt1
    | 
    | if(cargado==1)
    |     if ( xl>(xObjetivo-2) ) 
    |         Vt1 = 0;
    |     elseif ( xl>(xObjetivo-6) )
    |         Vt1 = VtMax/18;
    |     elseif ( xl>(xObjetivo-10) )
    |         Vt1 = VtMax/13;
    |     elseif ( xl>(xObjetivo-14) )
    |         Vt1 = VtMax/10;
    |     elseif ( xl>(xObjetivo-20) )
    |         Vt1 = VtMax/7;
    |     end
    | elseif(cargado==0)
    |     if ( xl>(xObjetivo-1.5) )  
    |         Vt1 = 0;
    |     elseif ( xl>(xObjetivo-4) ) 
    |         Vt1 = VtMax/16;
    |     elseif ( xl>(xObjetivo-9) ) 
    |         Vt1 = VtMax/11;
    |     elseif ( xl>(xObjetivo-14) )
    |         Vt1 = VtMax/8;
    |     elseif ( xl>(xObjetivo-20) ) 
    |         Vt1 = VtMax/6;
    |     end
    | end
  function calculaVh1:
    | function calculaVh1 %Descenso de ida
    | 
    | if(cargado==1)
    |     if ( yl<(yObjetivo+2) )
    |         Vh1 = 0;
    |     end
    |     
    | elseif(cargado==0)
    |     if ( yl<(yObjetivo+2) )
    |         Vh1 = 0;
    |     elseif ( yl<(yObjetivo+5) )
    |         Vh1 = VhMax/2.3;
    |     elseif ( yl<(yObjetivo+8) )
    |         Vh1 = VhMax/1.8;
    |     end
    | end
  function calculaTrayectoria_2:
    | function calculaTrayectoria_2
    | 
    | xPartida       = xCarrilMuelle(carrilPartida); 
    | yPartida       = hContenedor + 1; %1m de seguridad
    | numCarrilBarco = [1 2 3 4 5 6 7 8 9 10 11 12 13 14 15 16 17];
    | 
    | %% Ymax
    | %Obstáculo más alto a alcanzar hasta carril objetivo (de más a la IZQUIERDA)
    | xYmax = 0; Ymax  = 15; carrilYmax = 1; %Considero que es SB
    |     for j=1:carrilObjetivo
    |         if (yCarrilBarco(j)>Ymax)
    |              Ymax = yCarrilBarco(j);
    |             xYmax = xCarrilBarco(j);
    |             carrilYmax = numCarrilBarco(j);
    |         end
    |     end
    | 
    | Ymax = Ymax + 2; %2m extra de seguridad
    | if cargado==1   % Suma altura de contenedor si está cargado
    |      Ymax=Ymax+hContenedor;
    | end
    | 
    | %% Izaje inicial
    | xIni = xCarrilBarco(carrilObjetivo);
    | deltaYcarril2    = zeros(1,carrilObjetivo-1);
    | % Barrido de carriles para ver cuál interfiere más en el recorrido
    | for i=1:(carrilObjetivo-1)
    |     distanciaXcarril = xIni-xCarrilBarco(i);
    |     tiempoCarril     = distanciaXcarril/VtMax;
    |     distanciaYcarril = tiempoCarril*VhMax;
    |     deltaYcarril2(i) = yCarrilBarco(i)-(distanciaYcarril+yObjetivo+hContenedor+2); %Comienza en yCarril+hCont+2
    | end
    | 
    | if cargado==1   % Suma altura de contenedor si está cargado (carga debe pasar por arriba de obstáculo)
    |      deltaYcarril2 = deltaYcarril2+hContenedor;
    | end
    | 
    | if isempty(deltaYcarril2)
    |     y_inicial2 = 2;
    | else
    |     y_inicial2 = max(deltaYcarril2)+2; %2m extra de seguridad
    | end
    | 
    | if y_inicial2<0 
    |     y_inicial2 = 2;
    | end
    | 
    | %% Traslación exclusiva
    | x_inicial2 = 0;
    | % Barrido carriles para ver cual interfiere más en el recorrido
    | if(carrilYmax>1)
    |     deltaYcarril22    = zeros(1,(carrilYmax-1) );
    |     for i=1:(carrilYmax-1)
    |         deltaYcarril22(i)    = -100;
    |     end
    |     
    |     for i=1:(carrilYmax-1)
    |         distanciaXcarril  = xYmax-xCarrilBarco(i);
    |         tiempoCarril      = distanciaXcarril/VtMax;
    |         distanciaYcarril  = tiempoCarril*VhMax;
    |         hYcarril          = Ymax - distanciaYcarril;
    |         deltaYcarril22(i) = yCarrilBarco(i)-hYcarril;
    |     end
    |     
    |     if isempty(deltaYcarril22)
    |         MAXdeltaY = 0
    |     else
    |         MAXdeltaY = max(deltaYcarril22)
    |     end
    |     
    |     deltaYdeseada = 3; %3m de seguridad
    |     if cargado==1   % Suma altura de contenedor si está cargado
    |         deltaYdeseada = deltaYdeseada+hContenedor;
    |     end
    |     
    |     deltaReal = deltaYdeseada+MAXdeltaY;
    |     if(deltaReal<0)
    |         deltaReal=0;
    |     end
    |     
    |     tMAXdeltaY = deltaReal/VhMax
    |     distanciatMAX = tMAXdeltaY*VtMax;
    |     x_inicial2 = distanciatMAX+6; 
    | end 
    | 
    | if ( (xObjetivo-xPartida)<25 ) 
    |     x_inicial2 = x_inicial2 + (xObjetivo-xPartida) + 6
    | end
    | 
    | if cargado==1   % Suma altura de contenedor si está cargado
    |      yPartida   = yPartida   + hContenedor;
    | end
    | 
    | Ymax
    | xYmax
    | carrilYmax
    | y_inicial2
    | x_inicial2
    | xObjetivo
    | xPartida
  function calculaVt1_2:
    | function calculaVt1_2
    | 
    | if(cargado==1)
    |     if ( xl<(xPartida+2) )
    |         Vt1 = 0;
    |     elseif ( xl<(xPartida+6) )
    |         Vt1 = -VtMax/18;
    |     elseif ( xl<(xPartida+10) )
    |         Vt1 = -VtMax/13;
    |     elseif ( xl<(xPartida+14) )
    |         Vt1 = -VtMax/10;
    |     elseif ( xl<(xPartida+20) )
    |         Vt1 = -VtMax/7;
    |     end
    | elseif(cargado==0)
    |     if ( xl<(xPartida+1.5) )
    |         Vt1 = 0;
    |     elseif ( xl<(xPartida+4) )
    |         Vt1 = -VtMax/16;
    |     elseif ( xl<(xPartida+9) )
    |         Vt1 = -VtMax/11;
    |     elseif ( xl<(xPartida+14) ) 
    |         Vt1 = -VtMax/8;
    |     elseif ( xl<(xPartida+20) ) 
    |         Vt1 = -VtMax/6;
    |     end
    | end
  function calculaVh1_2:
    | function calculaVh1_2 %Descenso de vuelta
    | 
    | if(cargado==1)
    |     if ( yl<(yPartida+2) )
    |         Vh1 = 0;
    |     end
    | elseif(cargado==0)
    |     if ( yl<(yPartida+2) )
    |         Vh1 = 0;
    |     elseif ( yl<(yPartida+5) )
    |         Vh1 = VhMax/2.3;
    |     elseif ( yl<(yPartida+8) )
    |         Vh1 = VhMax/1.8;
    |     end
    | end
  function Vt1_manual:
    | function Vt1_manual
    | 
    | if( (pVt<0.2)&&(pVt>-0.2) )
    |     Vt1 = 0;
    | else
    |     Vt1 = pVt*VtMax/3;
    | end
  function Vh1_manual:
    | function Vh1_manual %Descenso de ida
    |  
    |  if( (pVh<0.2)&&(pVh>-0.2) )
    |      Vh1 = 0;
    |  else
    |      Vh1 = pVh*VhMax/3;
    | 
    | % if(pVh<0)
    | %     Vh1 = -VhMax/3;;
    | % elseif(pVh>0)
    | %     Vh1 = +VhMax/3;;   
    | % else
    | %     Vh1 = 0;
    | 
    | end
  function calculaCarrilActual:
    | function calculaCarrilActual 
    | 
    |     if(lado==1) % LADO BARCO
    |                     for x=5:5:50
    |                         if(xt>=(x-1.5) )
    |                             aux = (x+5)*(cantidadCarrilesBarco+1)/55 ;
    |                             carrilActual = uint8(aux);%+1)
    |                         end
    |                     end
    |     
    |     elseif(lado==0)
    |                     if    ( xt>=(-5) )  
    |                         carrilActual = uint8(6);
    |                     elseif(xt>=-10) 
    |                         carrilActual = uint8(5);
    |                     elseif(xt>=-15) 
    |                         carrilActual = uint8(4);
    |                     elseif(xt>=-20) 
    |                         carrilActual = uint8(3);
    |                     elseif(xt>=-25) 
    |                         carrilActual = uint8(2);
    |                     else %if(xt>=-30)
    |                         carrilActual = uint8(1);
    |                     end
    |     end
    |     %carrilActual
    | end

== matlab function Proyecto_Global_AyCD_Ultimo/ Planta/Cálculo Cable ==
  data: l output; xl input; yl input; xt input; Tita output; yt0 input
function [l,Tita]= calculoCable(xl,yl,xt,yt0)
    a    = xl-xt;
    b    = yt0-yl;
    l    = sqrt  ( a^2+b^2 );
    Tita = atan2 ( a,b );
end

== stateflow chart Proyecto_Global_AyCD_Ultimo/GRAFICO ==
  state GRAFICO [parallel]
    entry:
    contadorGrafico = 0;
    xtAnt = xt; xlAnt = xl; ylAnt = yl;
    during:
    graficoInstantaneo();
    settings: executionOrder=1
  state REVISION [parallel]
    settings: executionOrder=5
    state DESACTIVADA
      entry:
      graficoRevision();
    state ACTIVADA
      entry:
      graficoRevision();
    (default) -> REVISION.DESACTIVADA
    REVISION.DESACTIVADA -> REVISION.ACTIVADA : [revision==1]
    REVISION.ACTIVADA -> REVISION.DESACTIVADA : [revision==0]
  state ALARMA [parallel]
    settings: executionOrder=4
    state DESACTIVADA
      entry:
      graficoAlarma();
    state ACTIVADA
      entry:
      graficoAlarma();
    (default) -> ALARMA.DESACTIVADA
    ALARMA.DESACTIVADA -> ALARMA.ACTIVADA : [alarma==1]
    ALARMA.ACTIVADA -> ALARMA.DESACTIVADA : [alarma==0]
  state BALANCEO [parallel]
    settings: executionOrder=2
    state DESACTIVADO
      entry:
      graficoBalanceo();
    state ACTIVADO
      entry:
      graficoBalanceo();
    (default) -> ACTIVADO
    DESACTIVADO -> ACTIVADO : [balanceo==1]
    ACTIVADO -> DESACTIVADO : [balanceo==0]
  state SPREADER [parallel]
    settings: executionOrder=3
    state CARGADO
      entry:
      graficoSpreader();
    state VACIO
      entry:
      graficoSpreader();
    (default) -> VACIO
    VACIO -> CARGADO : [cargado==1]
    CARGADO -> VACIO : [cargado==0]
  data: xt input; xl input; yl input; alarma input; balanceo input; cargado input; xtAnt local; xlAnt local; ylAnt local; contadorGrafico local; revision input
  function graficoInicial:
    | function graficoInicial
    | 
    | figure(1)
    | MUELLE =[-35 -1 -1 -35 -35;0 0 -20 -20 0];   plot2d_green(MUELLE); hold on;
    | BARCO  =[0 0 50 50;15 -20.4 -20.4 15];       plot2d_red(BARCO);    hold on
    | VIGA   =[-30 50;45 45];                      plot2d_cyan(VIGA);    hold on;
    | 
    | %% Grafica contenedores iniciales  
    | for i=2:cantidadCarrilesBarco
    |     rayai = [xCarrilBarco(i)-bContenedor/2     xCarrilBarco(i)+bContenedor/2; -20 -20];
    |     plot2d_blue(rayai);   hold on;
    |     for j=1:nRand(i)
    |         CONTENEDORi = [xCarrilBarco(i)-bContenedor/2     xCarrilBarco(i)-bContenedor/2   xCarrilBarco(i)+bContenedor/2   xCarrilBarco(i)+bContenedor/2 ;
    |                       (j-1)*hContenedor-20    j*hContenedor-20      j*hContenedor-20     (j-1)*hContenedor-20  ];
    |         plot2d_blue(CONTENEDORi);   hold on;
    |     end
    | end
    | for i=-30:5:-5
    |         MUELLEi = [i-bContenedor/2     i-bContenedor/2   i+bContenedor/2   i+bContenedor/2 i-bContenedor/2;
    |                        0       hContenedor       hContenedor       0     0  ];
    |         plot2d_blue(MUELLEi);   hold on;
    | end
    | %text(-30,-10,' VACIO ','Color','red','FontSize',14)
    | 
    | %% Ymax
    | % x1=0;  x2=50;
    | % y1=34.5; y2=34.5;
    | % line([x1 x2],[y1 y2],'LineWidth',0.8,'color','magenta')
    | % 
    | % %% xYmax
    | % x1=10;  x2=10;
    | % y1=-20; y2=34.5;
    | % line([x1 x2],[y1 y2],'LineWidth',0.8,'color','magenta')
    | 
    | %% Grafica líneas de traslación simulatánea de subida -> (IDA)
    | % x1=-25;             x2=40;
    | % y1=3/8*x1+11.875;   y2=3/8*x2+11.875;
    | % line([x1 x2],[y1 y2],'LineWidth',0.8,'color','magenta')
    | %  
    | % x1=-25;                    x2=40;
    | % y1=3/8*x1+11.875+18.875;   y2=3/8*x2+11.875+18.875;
    | % line([x1 x2],[y1 y2],'LineWidth',0.8,'color','magenta')
    | % 
    | % %% Grafica lineas de traslación simulatánea de bajada ->
    | % for b=26:2:52
    | %     xx = [-30 50];
    | %     yy = [b -1.5/4*50+b];
    | %     line(xx,yy,'LineWidth',0.5,'color','cyan')
    | % end
  function graficoInstantaneo:
    | function graficoInstantaneo()
    | rectangle('Position',[-2,0,2,45],'FaceColor','y')%columna 2 rigida
    | contadorGrafico=contadorGrafico+1;
    | if (contadorGrafico==60)
    |     contadorGrafico=0;
    |     
    |     %Cable
    |     line([xlAnt  xtAnt],[ylAnt  44.5],'LineWidth',0.8,'color','white'); 
    |     line([xl     xt]   ,[yl     44.5],'LineWidth',0.5);
    |     
    |     %Carga
    |     plot(xlAnt,ylAnt,'w','MarkerSize',2,'MarkerFaceColor','w');
    |     plot(xl   ,   yl,'k','MarkerSize',2,'MarkerFaceColor','k');
    |     if(cargado==1)
    |     plot(xlAnt,ylAnt,'-s',...
    |     'LineWidth',2,...
    |     'MarkerSize',10,...
    |     'MarkerEdgeColor','white')
    |     plot(xl,yl,'-s',...
    |     'LineWidth',2,...
    |     'MarkerSize',10,...
    |     'MarkerEdgeColor','red')
    |     end
    |     if(cargado==0)
    |     plot(xlAnt,ylAnt,'-s',...
    |     'LineWidth',2,...
    |     'MarkerSize',10,...
    |     'MarkerEdgeColor','white')
    |     plot(xl,yl,'v',...
    |     'LineWidth',1,...
    |     'MarkerSize',1,...
    |     'MarkerEdgeColor','k',...
    |     'MarkerFaceColor',[0.1,0.1,0.1])
    |     end
    |     %Guarda valores anteriores para borrarlos en la próxima iteración
    |     xtAnt = xt; xlAnt = xl; ylAnt = yl;
    | end
    |  
    | 
    | end
  function graficoSpreader:
    | function graficoSpreader
    | 
    |     if (cargado == 0 )
    |         plot(-10,-11,'or','MarkerSize',10,'MarkerFaceColor','r'); 
    |         %%rectangle('Position',[-10 -41 2 2],'Curvature',[1 1],'FaceColor','r'):
    |         
    |     elseif(cargado == 1)
    |         plot(-10,-11,'og','MarkerSize',10,'MarkerFaceColor','g'); 
    |       
    |         
    |     end
    |     
    | end
  function graficoBalanceo:
    | function graficoBalanceo
    | 
    |     if (balanceo == 0 )
    |         plot(-10,-15,'or','MarkerSize',10,'MarkerFaceColor','r'); 
    |     elseif(balanceo == 1)
    |         plot(-10,-15,'og','MarkerSize',10,'MarkerFaceColor','g'); 
    |     end
    |     
    | end
  function graficoAlarma:
    | function graficoAlarma
    | 
    |     if (alarma == 0 )
    |         plot(-10,-7,'og','MarkerSize',10,'MarkerFaceColor','g'); 
    |     elseif(alarma == 1)
    |         plot(-10,-7,'or','MarkerSize',10,'MarkerFaceColor','r'); 
    |     end
    |     
    | end
  function graficoRevision:
    | function graficoRevision
    | 
    |     if (revision == 0 )
    |         plot(-10,-3,'og','MarkerSize',10,'MarkerFaceColor','g'); 
    |     elseif(revision == 1)
    |         plot(-10,-3,'or','MarkerSize',10,'MarkerFaceColor','r'); 
    |     end
    |     
    | end

== stateflow chart Proyecto_Global_AyCD_Ultimo/Nivel 0 ==
  state NORMAL
    entry: Vh0=0; Vt0=0; Revision = 0;
    state SITUACION_NORMAL
      entry:
      Alarma=0;
    state EMERGENCIA_FIN_CARRERA
      entry:
      Alarma=1;
    state EMERGENCIA_PULSADOR
      entry:
      Alarma=1;
    state EMERGENCIA_SOBREVELOCIDAD
      entry:
      Alarma=1;
    (default) -> SITUACION_NORMAL
    SITUACION_NORMAL -> EMERGENCIA_FIN_CARRERA [order 1] : [(fcL0==1)||(fcR0==1)]
    SITUACION_NORMAL -> EMERGENCIA_FIN_CARRERA [order 5] : [(fcU0==1)||(fcD0==1)]
    SITUACION_NORMAL -> EMERGENCIA_PULSADOR [order 3] : [pEmergencia==1]
    SITUACION_NORMAL -> EMERGENCIA_SOBREVELOCIDAD [order 4] : [ (Dlh>VhMax*1.1) || (Dlh<-VhMax*1.1) ]
    SITUACION_NORMAL -> EMERGENCIA_SOBREVELOCIDAD [order 2] : [ (Dxt>VtMax*1.1)  ||  (Dxt<-VtMax*1.1) ]
  state EMERGENCIA
    entry: Revision = 1;
    Vt0=0; Vh0=0;
    state MANUAL_EMERGENCIA
      during:
      calculaVt0_emergencia();
      calculaVh0_emergencia();
    state APAGAR_ALARMA
      entry:
      Vt0=0; Vh0=0; Alarma=0;
    (default) -> MANUAL_EMERGENCIA
    MANUAL_EMERGENCIA -> APAGAR_ALARMA : [pRevision==1]
  (default) -> NORMAL
  NORMAL -> EMERGENCIA : [Alarma==1]
  EMERGENCIA -> NORMAL : [Alarma==0]
  data: fcL0 input; fcR0 input; fcU0 input; fcD0 input; Vh0 output double; Vt0 output double; Dxt input; Dlh input; pVh input; pVt input; pRevision input; pEmergencia input; VtMax input; VhMax input; Revision output double; Alarma output double
  function calculaVt0_emergencia:
    | function calculaVt0_emergencia
    | 
    | if(   ((pVt>0.2)&&(fcR0==0)) || ((pVt<-0.2)&&(fcL0==0)) )
    |      Vt0 = pVt*VtMax/3;
    | else
    |      Vt0 = 0;
    | end
  function calculaVh0_emergencia:
    | function calculaVh0_emergencia %Descenso de ida
    | 
    | if( ((pVh>0.2)&&(fcD0==0)) || ((pVh<-0.2)&&(fcU0==0)) )
    |     Vh0 = pVh*VhMax/3;
    | else
    |     Vh0 = 0;
    | end
    | 
    | if ( (fcR0==0)&&(fcL0==0)&&(fcU0==0)&&(fcD0==0) )
    |     Revision = 0;
    | else 
    |     Revision = 1;
    | end
